simulink model "embedded_persistent"  (Simulink 7.6)
settings: Solver=FixedStepDiscrete  StartTime=0.0  StopTime=10.0  FixedStep=1  RelTol=1e-3
PreLoadFcn:
  | simpleBus
settings Model: Creator=Harmon S. Nine  LastModifiedBy=c2wt
settings DataIOCC: SignalLogging=off  DSMLogging=off
settings DebuggingCC: StrictBusMsg=Warning
settings SFSimCC: SimParseCustomCode=off

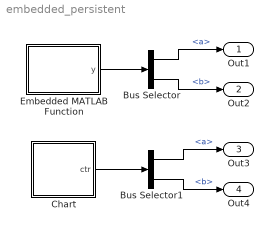
== system embedded_persistent ==
  Bus Selector : BusSelector  OutputSignals=a,b
  Bus Selector1 : BusSelector  OutputSignals=a,b
  Chart : Stateflow chart  TreatAsAtomicUnit=on
  Embedded MATLAB Function : Stateflow chart  TreatAsAtomicUnit=on
  Out1 : Outport
  Out2 : Outport  Port=2
  Out3 : Outport  Port=3
  Out4 : Outport  Port=4
  wires:
  Bus Selector/2 -> Out2/1  "<b>"
  Bus Selector/1 -> Out1/1  "<a>"
  Embedded MATLAB Function/1(y) -> Bus Selector/1
  Bus Selector1/1 -> Out3/1  "<a>"
  Bus Selector1/2 -> Out4/1  "<b>"
  Chart/1(ctr) -> Bus Selector1/1

== stateflow chart Chart ==
  state state1
    en: ctr = getCtr();
  state1 -> state1
  (default) -> state1
  data: out function_output Bus: simpleBus; ctr output Bus: simpleBus
  function out = getCtr:
    | function out = getCtr()
    | %#eml
    | 
    | persistent x;
    | 
    | if isempty(x)
    |     x = struct('a', 1, 'b', -1 );
    | end
    | 
    | x.a = x.a + 2;
    | x.b = x.b - 2;
    | 
    | out = x;

== matlab function Embedded MATLAB Function ==
  data: y output Bus: simpleBus
function y = fcn()
%#eml

persistent x;

if isempty(x)
  x.a = 0;
  x.b = 0;
end

x.a = x.a + 1;
x.b = x.b - 1;
y = x;
